simulink model "sustainATHON"  (R2020a)
settings: Solver=ode8  StartTime=0.0  StopTime=20000  RelTol=1e-3
values from neighbouring files (symbols this model uses):
  c = 1005.4    [cal_sustainathon.m]
  cost = 0.09/3.6e6    (= 2.5e-08)    [cal_sustainathon.m]
  M = (length*width*height)*densAir    (= 49000)    [cal_sustainathon.m]
  Mdot = 10    [cal_sustainathon.m]
  Req = RWall*RWindow*10/(RWall + RWindow)    (= 0.000211783641832)    [cal_sustainathon.m]
undefined symbols (not defined in the file or in its folder): TinIC
libraries: simulink x6, dspstat3 x1
settings Model: Creator=Amogh Kuruwatti  LastModifiedBy=Amogh Kuruwatti

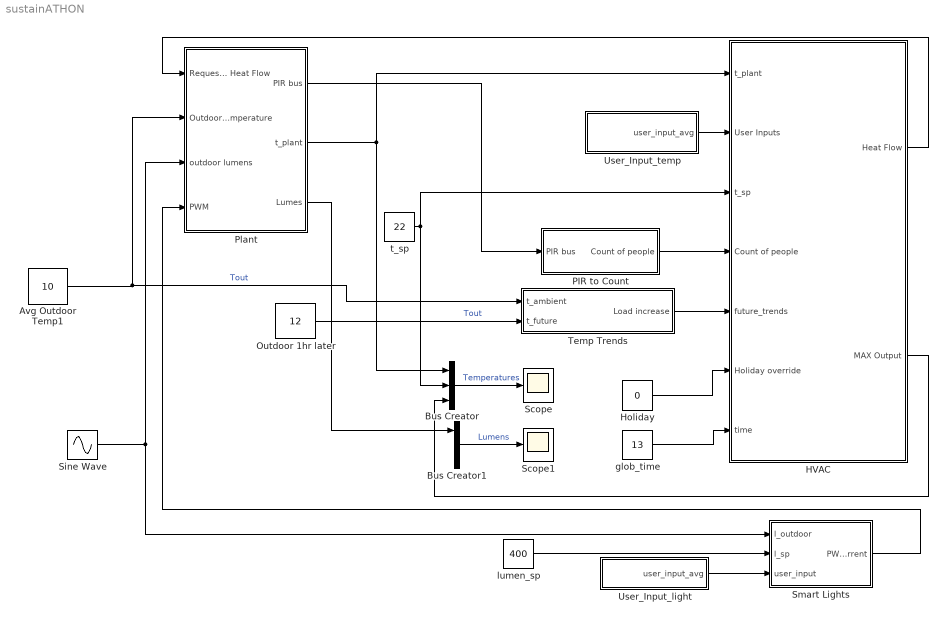
== system sustainATHON ==
  Avg Outdoor Temp1 : Constant  Value=10  SampleTime=-1
  Bus Creator : BusCreator  Inputs=3
  Bus Creator1 : BusCreator  Inputs=3
  HVAC : Subsystem
  Holiday : Constant  Value=0  SampleTime=-1
  Outdoor 1hr later : Constant  Value=12  SampleTime=-1
  PIR to Count : Subsystem
  Plant : Subsystem
  Scope : Scope
  Scope1 : Scope
  Sine Wave : Sin  Amplitude=100  Frequency=0.001  SampleTime=0
  Smart Lights : Subsystem
  Temp Trends : Subsystem
  User_Input_light : Subsystem
  User_Input_temp : Subsystem
  glob_time : Constant  Value=13  SampleTime=-1
  lumen_sp : Constant  Value=400
  t_sp : Constant  Value=22  SampleTime=-1
  wires:
  User_Input_temp/1(user_input_avg) -> HVAC/2(User Inputs)
  Plant/1(PIR bus) -> PIR to Count/1(PIR bus)
  Plant/2(t_plant) -> HVAC/1(t_plant), Bus Creator/1
  HVAC/1(Heat Flow) -> Plant/1(Request Heat Flow)
  Holiday/1 -> HVAC/6(Holiday override)
  glob_time/1 -> HVAC/7(time)
  Bus Creator/1 -> Scope/1  "Temperatures"
  Temp Trends/1(Load increase) -> HVAC/5(future_trends)
  PIR to Count/1(Count of people) -> HVAC/4(Count of people)
  User_Input_light/1(user_input_avg) -> Smart Lights/3(user_input)
  lumen_sp/1 -> Smart Lights/2(l_sp)
  Sine Wave/1 -> Smart Lights/1(l_outdoor), Plant/3(outdoor lumens)
  Outdoor 1hr later/1 -> Temp Trends/2(t_future)  "Tout"
  t_sp/1 -> Bus Creator/2, HVAC/3(t_sp)
  HVAC/2(MAX Output) -> Bus Creator/3
  Avg Outdoor Temp1/1 -> Temp Trends/1(t_ambient), Plant/2(Outdoor Temperature)  "Tout"
  Bus Creator1/1 -> Scope1/1  "Lumens"
  Smart Lights/1(PWM Current) -> Plant/4(PWM)
  Plant/3(Lumes) -> Bus Creator1/1

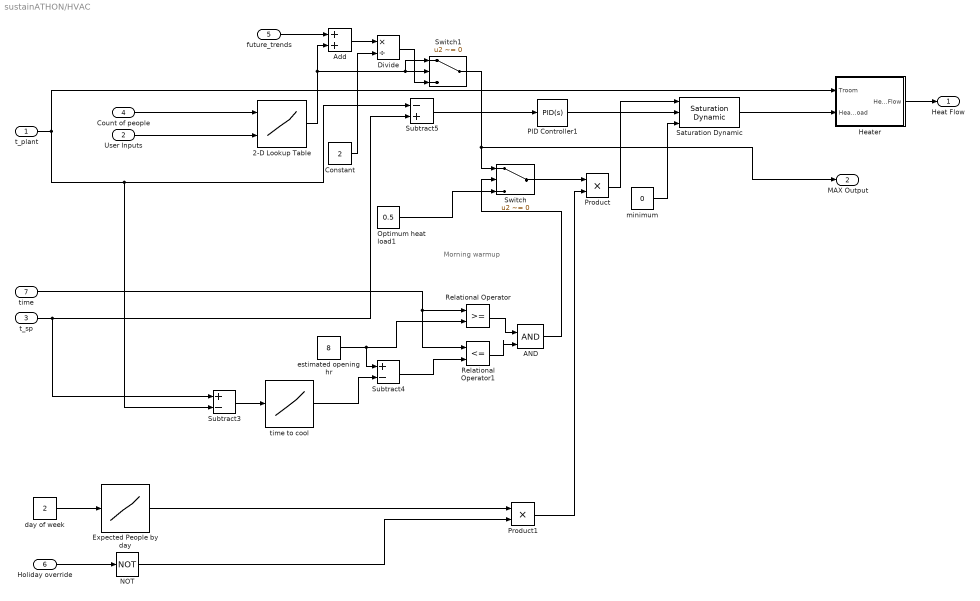
== system sustainATHON/HVAC ==
  note: Morning warmup
  t_plant : Inport
  User Inputs : Inport  Port=2
  t_sp : Inport  Port=3
  Count of people : Inport  Port=4
  future_trends : Inport  Port=5
  Holiday override : Inport  Port=6
  time : Inport  Port=7
  2-D Lookup Table : Lookup_n-D  BreakpointsForDimension1=[0 200 400 600 800 1000]  BreakpointsForDimension2=[-1 -0.75 -0.5 -0.25 0 0.25 0.5 0.75 1]  Table=[ 0 0 0 0 0 0 0 0 0 ; -0.4 -0.3 -0.2 -0.1 0 0.1 0.2 0.3 0.4 ; -0.8 -0.6 -0.4 -0.2 0 0.2 0.4 0.6 0.8;-1 -1 -0.66 -0.33 0 0.33 0.66 1 1; -1 -1 -1 -0.5 0 0.5 1 1 1; -1 -1 -1 -1 0 1 1 1 1 ]  InternalRulePriority=Speed  RndMeth=Simplest  InputSameDT=on
  AND : Logic  IconShape=distinctive  AllPortsSameDT=off  OutDataTypeStr=boolean
  Add : Sum
  Constant : Constant  Value=2  SampleTime=-1
  Divide : Product  Inputs=*/
  Expected People by day : Lookup_n-D  NumberOfTableDimensions=1  LookupTableObject=''  BreakpointsForDimension1=[1:7]  BreakpointsForDimension1FirstPoint=7  BreakpointsForDimension2FirstPoint=10  BreakpointsForDimension2Spacing=12  IndexSearchMethod=Evenly spaced points  Table=[0 1 1 1 1 1 1]  InterpMethod=Flat  DiagnosticForOutOfRangeInput=Error  InternalRulePriority=Speed  RndMeth=Simplest  InputSameDT=on
  Heater : Subsystem
  NOT : Logic  Operator=NOT  IconShape=distinctive  AllPortsSameDT=off  OutDataTypeStr=boolean
  Optimum heat load1 : Constant  Value=0.5  SampleTime=-1
  PID Controller1 : simulink/Continuous/PID Controller  Controller=PID  Form=Parallel  TimeDomain=Continuous-time  UseExternalTs=off  SampleTime=-1  IntegratorMethod=Forward Euler  FilterMethod=Forward Euler  ControllerParametersSource=internal  P=10  I=0  D=0  UseFilter=on  N=100  TunerSelectOption=Transfer Function Based (PID Tuner App)  InitialConditionSource=internal  InitialConditionForIntegrator=0  InitialConditionForFilter=0  DifferentiatorICPrevScaledInput=0  ExternalReset=none  TrackingMode=off  Kt=1  LimitOutput=off  UpperSaturationLimit=inf  LowerSaturationLimit=-inf  LinearizeAsGain=on  AntiWindupMode=none  Kb=1  POutMin=[]  POutMax=[]  IOutMin=[]  IOutMax=[]  DOutMin=[]  DOutMax=[]  NOutMin=[]  NOutMax=[]  SumOutMin=[]  SumOutMax=[]  SaturationOutMin=[]  SaturationOutMax=[]  PParamMin=[]  PParamMax=[]  IParamMin=[]  IParamMax=[]  DParamMin=[]  DParamMax=[]  NParamMin=[]  NParamMax=[]  KbParamMin=[]  KbParamMax=[]  KtParamMin=[]  KtParamMax=[]  KbOutMin=[]  KbOutMax=[]  KtOutMin=[]  KtOutMax=[]  IntegratorOutMin=[]  IntegratorOutMax=[]  FilterOutMin=[]  FilterOutMax=[]  SumI1OutMin=[]  SumI1OutMax=[]  SumI2OutMin=[]  SumI2OutMax=[]  SumI3OutMin=[]  SumI3OutMax=[]  SumI4OutMin=[]  SumI4OutMax=[]  SumDOutMin=[]  SumDOutMax=[]  DifferentiatorOutMin=[]  DifferentiatorOutMax=[]  FilterDiffOutCoefMin=[]  FilterDiffOutCoefMax=[]  ReciprocalOutMin=[]  ReciprocalOutMax=[]  SumDenOutMin=[]  SumDenOutMax=[]  SumNumOutMin=[]  SumNumOutMax=[]  DivideOutMin=[]  DivideOutMax=[]  UdiffTsProdOutMin=[]  UdiffTsProdOutMax=[]  NTsProdOutMin=[]  NTsProdOutMax=[]  UintegralTsProdOutMin=[]  UintegralTsProdOutMax=[]  UngainTsProdOutMin=[]  UngainTsProdOutMax=[]  IntegratorContinuousStateAttributes=''  IntegratorStateMustResolveToSignalObject=off  IntegratorRTWStateStorageClass=Auto  FilterContinuousStateAttributes=''  FilterStateMustResolveToSignalObject=off  FilterRTWStateStorageClass=Auto  ParallelPVariant=InternalParameters  IdealPVariant=Disabled  IVariant=InternalParameters  DVariant=InternalParameters  IntegratorVariant=Continuous  SatVariant=Disabled  AWVariant=Passthrough  PCopyVariant=Disabled  TRVariant=Disabled  FdbkBlocksVariant=Forward  IdealPFdbkVariant=Disabled  SatFdbkVariant=Disabled  DerivativeFilterVariant=ContFilter  NVariant=InternalParameters  NCopyVariant=Disabled  FilterICVariant=InternalICsFilter  IntegratorICVariant=InternalICs  ExternalResetVariant=Disabled  TRSumVariant=Passthrough  SumFdbkVariant=Disabled  SumVariant=Sum_PID  TsampFilterVariant=InternalTs  TsampNgainVariant=Passthrough  TsampIntegralVariant=Passthrough
  Product : Product
  Product1 : Product
  Relational Operator : RelationalOperator  OutDataTypeStr=boolean  RndMeth=Simplest
  Relational Operator1 : RelationalOperator  Operator=<=  OutDataTypeStr=boolean  RndMeth=Simplest
  Saturation Dynamic : simulink/Discontinuities/Saturation Dynamic  OutMin=[]  OutMax=[]  OutDataTypeStr=Inherit: Same as second input  OutDataType=fixdt(1, 16)  OutScaling=2^-10  DoSatur=off
  Subtract3 : Sum  Inputs=+-
  Subtract4 : Sum  Inputs=+-
  Subtract5 : Sum  Inputs=-+
  Switch : Switch  Criteria=u2 ~= 0
  Switch1 : Switch  Criteria=u2 ~= 0
  day of week : Constant  Value=2  SampleTime=-1
  estimated opening hr : Constant  Value=8  SampleTime=-1
  minimum : Constant  Value=0  SampleTime=-1
  time to cool : Lookup_n-D  NumberOfTableDimensions=1  LookupTableObject=''  BreakpointsForDimension1=[-10:10]  BreakpointsForDimension1FirstPoint=7  BreakpointsForDimension2FirstPoint=10  BreakpointsForDimension2Spacing=12  IndexSearchMethod=Evenly spaced points  Table=[-4.7 -3.8 -3 -2.3 -1.7 -1.2 -0.8 -0.5 -0.25 -0.1 0 0.1 0.25 0.5 0.8 1.2 1.7 2.3 3 3.8 4.7]  InterpMethod=Flat  DiagnosticForOutOfRangeInput=Error  InternalRulePriority=Speed  RndMeth=Simplest  InputSameDT=on
  Heat Flow : Outport
  MAX Output : Outport  Port=2
  wires:
  t_sp/1 -> Subtract5/2, Subtract3/1
  2-D Lookup Table/1 -> Switch1/1, Switch1/2, Add/2
  Constant/1 -> Divide/2
  Count of people/1 -> 2-D Lookup Table/1
  future_trends/1 -> Add/1
  Add/1 -> Divide/1
  t_plant/1 -> Heater/1(Troom), Subtract3/2, Subtract5/1
  Expected People by day/1 -> Product1/1
  day of week/1 -> Expected People by day/1
  Holiday override/1 -> NOT/1
  NOT/1 -> Product1/2
  estimated opening hr/1 -> Relational Operator/2, Subtract4/1
  Subtract4/1 -> Relational Operator1/2
  time/1 -> Relational Operator/1, Relational Operator1/1
  Relational Operator/1 -> AND/1
  Relational Operator1/1 -> AND/2
  AND/1 -> Switch/2
  User Inputs/1 -> 2-D Lookup Table/2
  Subtract5/1 -> PID Controller1/1
  PID Controller1/1 -> Saturation Dynamic/2
  minimum/1 -> Saturation Dynamic/3
  Saturation Dynamic/1 -> Heater/2(Heat Load)
  Heater/1(HeatFlow) -> Heat Flow/1
  Product1/1 -> Product/2
  Switch/1 -> Product/1
  Product/1 -> Saturation Dynamic/1
  Optimum heat load1/1 -> Switch/3
  time to cool/1 -> Subtract4/2
  Subtract3/1 -> time to cool/1
  Divide/1 -> Switch1/3
  Switch1/1 -> MAX Output/1, Switch/1

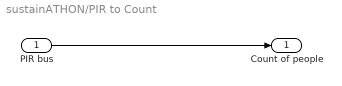
== system sustainATHON/PIR to Count ==
  PIR bus : Inport
  Count of people : Outport
  wires:
  PIR bus/1 -> Count of people/1

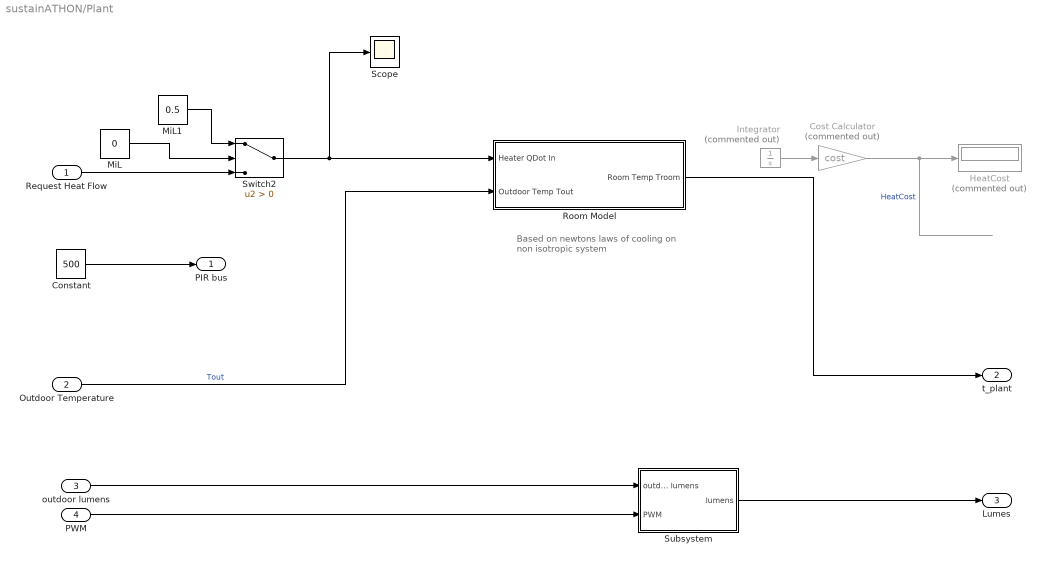
== system sustainATHON/Plant ==
  note: Based on newtons laws of cooling
      | on non isotropic system
  Request Heat Flow : Inport
  Outdoor Temperature : Inport  Port=2
  outdoor lumens : Inport  Port=3
  PWM : Inport  Port=4
  Constant : Constant  Value=500  SampleTime=-1
  Cost Calculator : Gain  Commented=on  Gain=cost  SaturateOnIntegerOverflow=on  OutDataTypeStr=Inherit: Same as input  ParamDataTypeStr=Inherit: Same as input
  HeatCost : Display  Commented=on
  Integrator : Integrator  Commented=on
  MiL : Constant  Value=0  SampleTime=-1
  MiL1 : Constant  Value=0.5  SampleTime=-1
  Room Model : Subsystem
  Scope : Scope
  Subsystem : Subsystem
  Switch2 : Switch  Criteria=u2 > Threshold
  PIR bus : Outport
  t_plant : Outport  Port=2
  Lumes : Outport  Port=3
  wires:
  Constant/1 -> PIR bus/1
  MiL/1 -> Switch2/2
  Request Heat Flow/1 -> Switch2/3
  MiL1/1 -> Switch2/1
  Outdoor Temperature/1 -> Room Model/2(Outdoor Temp Tout)  "Tout"
  Room Model/1(Room Temp Troom) -> t_plant/1
  Integrator/1 -> Cost Calculator/1
  Cost Calculator/1 -> HeatCost/1  "HeatCost"
  Switch2/1 -> Scope/1, Room Model/1(Heater QDot In)
  outdoor lumens/1 -> Subsystem/1(outdoor lumens)
  PWM/1 -> Subsystem/2(PWM)
  Subsystem/1(lumens) -> Lumes/1

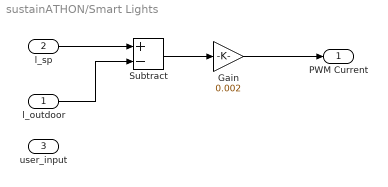
== system sustainATHON/Smart Lights ==
  l_outdoor : Inport
  l_sp : Inport  Port=2
  user_input : Inport  Port=3
  Gain : Gain  Gain=0.002
  Subtract : Sum  Inputs=+-
  PWM Current : Outport
  wires:
  l_sp/1 -> Subtract/1
  l_outdoor/1 -> Subtract/2
  Subtract/1 -> Gain/1
  Gain/1 -> PWM Current/1

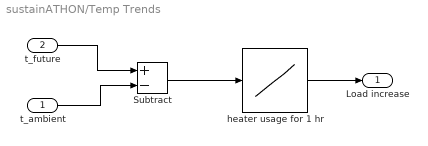
== system sustainATHON/Temp Trends ==
  t_ambient : Inport
  t_future : Inport  Port=2
  Subtract : Sum  Inputs=+-
  heater usage for 1 hr : Lookup_n-D  NumberOfTableDimensions=1  LookupTableObject=''  BreakpointsForDimension1=[-2 -1.5 -1 -0.5 0 0.5 1 1.5 2]  BreakpointsForDimension1FirstPoint=7  BreakpointsForDimension2FirstPoint=10  BreakpointsForDimension2Spacing=12  IndexSearchMethod=Evenly spaced points  Table=[-0.2 -0.15 -0.1 -0.05 0 0.05 0.1 0.15 0.2]  InterpMethod=Flat  DiagnosticForOutOfRangeInput=Error  InternalRulePriority=Speed  RndMeth=Simplest  InputSameDT=on
  Load increase : Outport
  wires:
  t_future/1 -> Subtract/1
  t_ambient/1 -> Subtract/2
  heater usage for 1 hr/1 -> Load increase/1
  Subtract/1 -> heater usage for 1 hr/1

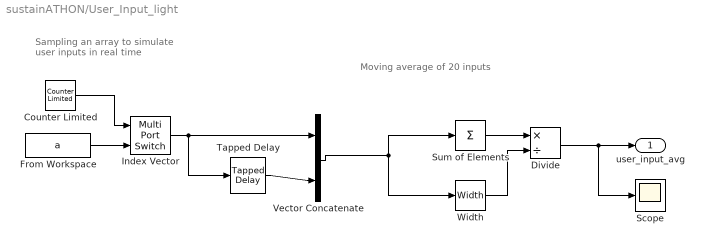
== system sustainATHON/User_Input_light ==
  note: Moving average of 20 inputs
  note: Sampling an array to simulate
      | user inputs in real time
  Counter Limited : simulink/Sources/Counter Limited  uplimit=70  tsamp=-1
  Divide : Product  Inputs=*/
  From Workspace : FromWorkspace  VariableName=a
  Index Vector : MultiPortSwitch  DataPortOrder=Zero-based contiguous  Inputs=1  zeroidx=on
  Scope : Scope
  Sum of Elements : Sum  Inputs=+
  Tapped Delay : simulink/Discrete/Tapped Delay  vinit=0.0  samptime=-1  NumDelays=20  DelayOrder=Oldest  includeCurrent=off
  Vector Concatenate : Concatenate
  Width : Width
  user_input_avg : Outport
  wires:
  Sum of Elements/1 -> Divide/1
  Width/1 -> Divide/2
  Tapped Delay/1 -> Vector Concatenate/2
  Vector Concatenate/1 -> Sum of Elements/1, Width/1
  Index Vector/1 -> Tapped Delay/1, Vector Concatenate/1
  From Workspace/1 -> Index Vector/2
  Counter Limited/1 -> Index Vector/1
  Divide/1 -> user_input_avg/1, Scope/1

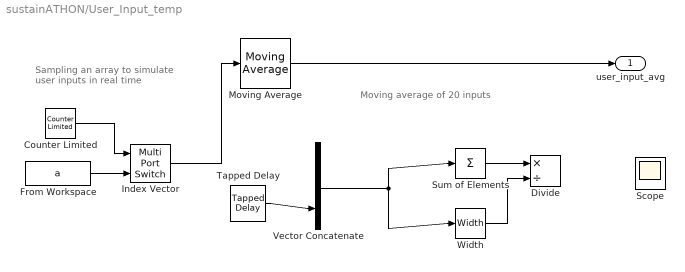
== system sustainATHON/User_Input_temp ==
  note: Moving average of 20 inputs
  note: Sampling an array to simulate
      | user inputs in real time
  Counter Limited : simulink/Sources/Counter Limited  uplimit=70  tsamp=-1
  Divide : Product  Inputs=*/
  From Workspace : FromWorkspace  VariableName=a
  Index Vector : MultiPortSwitch  DataPortOrder=Zero-based contiguous  Inputs=1  zeroidx=on
  Moving Average : dspstat3/Moving Average  Method=Sliding window  ForgettingFactorPort=off  SpecifyWindowLength=on  WindowLength=20  ForgettingFactor=0.9  SimulateUsing=Code generation
  Scope : Scope
  Sum of Elements : Sum  Inputs=+
  Tapped Delay : simulink/Discrete/Tapped Delay  vinit=0.0  samptime=-1  NumDelays=20  DelayOrder=Oldest  includeCurrent=off
  Vector Concatenate : Concatenate
  Width : Width
  user_input_avg : Outport
  wires:
  Sum of Elements/1 -> Divide/1
  Width/1 -> Divide/2
  Tapped Delay/1 -> Vector Concatenate/2
  Vector Concatenate/1 -> Sum of Elements/1, Width/1
  From Workspace/1 -> Index Vector/2
  Counter Limited/1 -> Index Vector/1
  Index Vector/1 -> Moving Average/1
  Moving Average/1 -> user_input_avg/1

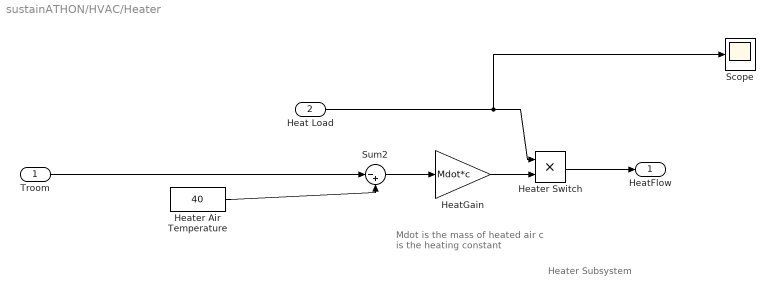
== system sustainATHON/HVAC/Heater ==
  note: Mdot is the mass of heated air
      | c is the heating constant
  note: Heater Subsystem
  Troom : Inport
  Heat Load : Inport  Port=2
  HeatGain : Gain  Gain=Mdot*c
  Heater Air Temperature : Constant  Value=40
  Heater Switch : Product  RndMeth=Zero
  Scope : Scope
  Sum2 : Sum  Inputs=|-+
  HeatFlow : Outport  VectorParamsAs1DForOutWhenUnconnected=off
  wires:
  Troom/1 -> Sum2/1
  Sum2/1 -> HeatGain/1
  Heat Load/1 -> Scope/1, Heater Switch/1
  HeatGain/1 -> Heater Switch/2
  Heater Air Temperature/1 -> Sum2/2
  Heater Switch/1 -> HeatFlow/1

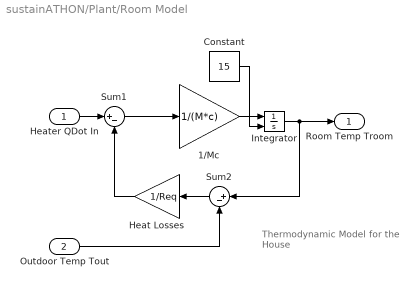
== system sustainATHON/Plant/Room Model ==
  note: Thermodynamic Model
      | for the House
  Heater QDot In : Inport
  Outdoor Temp Tout : Inport  Port=2
  1/Mc : Gain  Gain=1/(M*c)  SaturateOnIntegerOverflow=on  OutDataTypeStr=Inherit: Same as input  ParamDataTypeStr=Inherit: Same as input
  Constant : Constant  Value=15  SampleTime=-1
  Heat Losses : Gain  Gain=1/Req  SaturateOnIntegerOverflow=on  OutDataTypeStr=Inherit: Same as input  ParamDataTypeStr=Inherit: Same as input
  Integrator : Integrator  InitialConditionSource=external  InitialCondition=TinIC
  Sum1 : Sum  Inputs=|+-  InputSameDT=on  SaturateOnIntegerOverflow=on  OutDataTypeStr=Inherit: Same as first input
  Sum2 : Sum  Inputs=|+-  InputSameDT=on  SaturateOnIntegerOverflow=on  OutDataTypeStr=Inherit: Same as first input
  Room Temp Troom : Outport  InitialOutput=0  VectorParamsAs1DForOutWhenUnconnected=off
  wires:
  Outdoor Temp Tout/1 -> Sum2/2
  Heater QDot In/1 -> Sum1/1
  Sum1/1 -> 1/Mc/1
  Sum2/1 -> Heat Losses/1
  Heat Losses/1 -> Sum1/2
  1/Mc/1 -> Integrator/1
  Integrator/1 -> Sum2/1, Room Temp Troom/1
  Constant/1 -> Integrator/2

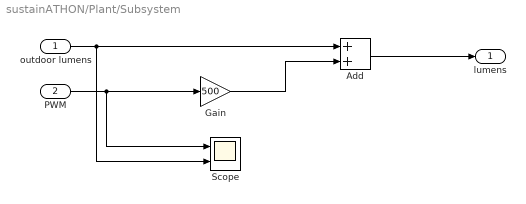
== system sustainATHON/Plant/Subsystem ==
  outdoor lumens : Inport
  PWM : Inport  Port=2
  Add : Sum
  Gain : Gain  Gain=500
  Scope : Scope  NumInputPorts=2
  lumens : Outport
  wires:
  Add/1 -> lumens/1
  PWM/1 -> Scope/1, Gain/1
  Gain/1 -> Add/2
  outdoor lumens/1 -> Add/1, Scope/2
